simulink model "modeloGago1"  (R2016a)
settings: Solver=VariableStepAuto  StartTime=0.0  StopTime=2000.0  FixedStep=0.001  RelTol=1e-3
values from neighbouring files (symbols this model uses):
  g = 9.82    [parametros.m]
  m = 6.165e3    (= 6165)    [parametros.m]
  thr = 167.97e3    (= 167970)    [parametros.m]
libraries: simulink x1
settings Model: Creator=raphaelbp12  LastModifiedBy=raphaelbp12
settings SolverCC: AutoInsertRateTranBlk=on

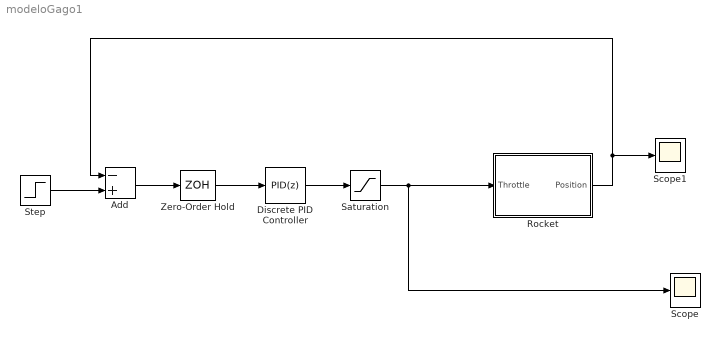
== system modeloGago1 ==
  Add : Sum  Inputs=-+
  Discrete PID Controller : simulink/Continuous/PID Controller  Controller=PID  TimeDomain=Discrete-time  SampleTime=1  IntegratorMethod=Forward Euler  FilterMethod=Forward Euler  Form=Parallel  UseFilter=on  ControllerParametersSource=internal  P=6.50338843681043e-07  I=3.15938846867281e-10  D=0.000315404958398162  N=0.0236954332278764  InitialConditionSource=internal  InitialConditionForIntegrator=0  InitialConditionForFilter=0  ExternalReset=none  LimitOutput=off  UpperSaturationLimit=inf  LowerSaturationLimit=-inf  LinearizeAsGain=off  AntiWindupMode=none  Kb=1  TrackingMode=off  Kt=1  PParamMin=[]  PParamMax=[]  IParamMin=[]  IParamMax=[]  DParamMin=[]  DParamMax=[]  NParamMin=[]  NParamMax=[]  KbParamMin=[]  KbParamMax=[]  KtParamMin=[]  KtParamMax=[]  POutMin=[]  POutMax=[]  IOutMin=[]  IOutMax=[]  DOutMin=[]  DOutMax=[]  NOutMin=[]  NOutMax=[]  KbOutMin=[]  KbOutMax=[]  KtOutMin=[]  KtOutMax=[]  IntegratorOutMin=[]  IntegratorOutMax=[]  FilterOutMin=[]  FilterOutMax=[]  SumOutMin=[]  SumOutMax=[]  SumI1OutMin=[]  SumI1OutMax=[]  SumI2OutMin=[]  SumI2OutMax=[]  SumI3OutMin=[]  SumI3OutMax=[]  SumDOutMin=[]  SumDOutMax=[]  SaturationOutMin=[]  SaturationOutMax=[]  IntegratorContinuousStateAttributes=''  IntegratorStateMustResolveToSignalObject=off  IntegratorRTWStateStorageClass=Auto  FilterContinuousStateAttributes=''  FilterStateMustResolveToSignalObject=off  FilterRTWStateStorageClass=Auto  DifferentiatorICPrevScaledInput=0  DifferentiatorOutMin=[]  DifferentiatorOutMax=[]
  Rocket : Subsystem
  Saturation : Saturate  UpperLimit=1  LowerLimit=0
  Scope : Scope
  Scope1 : Scope
  Step : Step  Time=0  After=2000  SampleTime=0
  Zero-Order Hold : ZeroOrderHold  SampleTime=0.001
  wires:
  Rocket/1(Position) -> Scope1/1, Add/1
  Step/1 -> Add/2
  Add/1 -> Zero-Order Hold/1
  Discrete PID Controller/1 -> Saturation/1
  Saturation/1 -> Scope/1, Rocket/1(Throttle)
  Zero-Order Hold/1 -> Discrete PID Controller/1

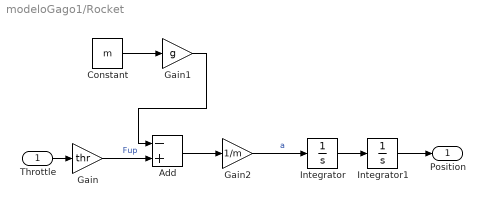
== system modeloGago1/Rocket ==
  Throttle : Inport
  Add : Sum  Inputs=-+
  Constant : Constant  Value=m
  Gain : Gain  Gain=thr
  Gain1 : Gain  Gain=g
  Gain2 : Gain  Gain=1/m
  Integrator : Integrator
  Integrator1 : Integrator
  Position : Outport
  wires:
  Integrator/1 -> Integrator1/1
  Integrator1/1 -> Position/1
  Gain/1 -> Add/2  "Fup"
  Throttle/1 -> Gain/1
  Constant/1 -> Gain1/1
  Gain1/1 -> Add/1
  Gain2/1 -> Integrator/1  "a"
  Add/1 -> Gain2/1
